simulink model "ControlSystem"  (R2015a)
settings: Solver=ode45  StartTime=0.0  StopTime=10.0  RelTol=1e-3
settings Model: Creator=pc  LastModifiedBy=pc

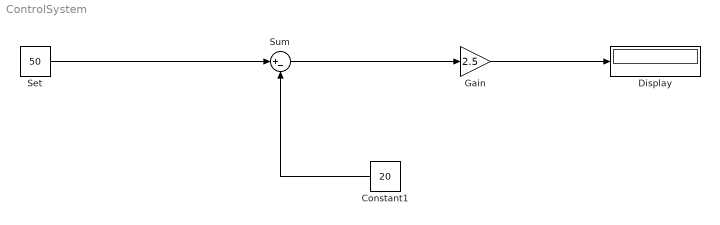
== system ControlSystem ==
  Constant1 : Constant  Value=20
  Display : Display
  Gain : Gain  Gain=2.5
  Set : Constant  Value=50
  Sum : Sum  Inputs=|+-
  wires:
  Set/1 -> Sum/1
  Sum/1 -> Gain/1
  Gain/1 -> Display/1
  Constant1/1 -> Sum/2
